simulink model "RespiratorPlantModel"  (R2018b)
settings: Solver=FixedStepAuto  StartTime=0.0  StopTime=30  FixedStep=0.001  MaxStep=0.001  RelTol=1e-3
values from neighbouring files (symbols this model uses):
  BTClockRemoval = 1    [RespiratorPlantModel_init.m]
  Cpoumon = 0.1    [RespiratorPlantModel_init.m]
  Dinttuy = 6    [RespiratorPlantModel_init.m]
  e = 4.5    [RespiratorPlantModel_init.m]
  hlibtuy = 0.05    [RespiratorPlantModel_init.m]
  Patm = 0    [RespiratorPlantModel_init.m]
  Rex = 12.5    [RespiratorPlantModel_init.m]
  Rpoumon = 15    [RespiratorPlantModel_init.m]
  tinsp = 1    [RespiratorPlantModel_init.m]
  X_makair = [0 1.428571429 2.857142857 4.285714286 5.714285714 7.142857143 8.571428571 10 11.42857143 12.85714286 14.28571429 15.71428571 ... (33 elements, 1x33)]    [X_makair.mat]
  Y_makair = [2730.624562 2737.5 2745.890411 2823.971473 2900.599169 3000.432167 3171.512706 3284.514664 3433.346305 3592.109976 3939.708667 4053.269029 ... (33 elements, 1x33)]    [Y_makair.mat]
libraries: simulink x8, simulink_extras x1
settings Model: Creator=FASSI  LastModifiedBy=VITIE
settings SolverCC: AlgebraicLoopSolver=LineSearch

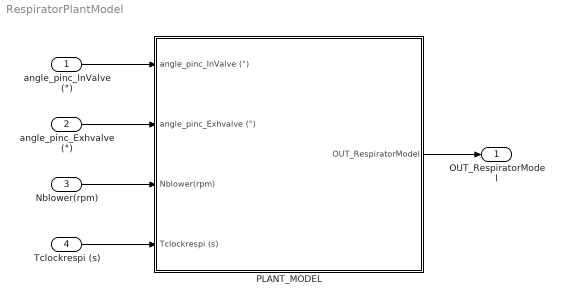
== system RespiratorPlantModel ==
  angle_pinc_InValve (°) : Inport
  angle_pinc_Exhvalve (°) : Inport  Port=2
  Nblower(rpm) : Inport  Port=3
  Tclockrespi (s) : Inport  Port=4
  PLANT_MODEL : Subsystem
  OUT_RespiratorModel : Outport  OutDataTypeStr=Bus: Respirator
  wires:
  angle_pinc_Exhvalve (°)/1 -> PLANT_MODEL/2(angle_pinc_Exhvalve (°))
  angle_pinc_InValve (°)/1 -> PLANT_MODEL/1(angle_pinc_InValve (°))
  Nblower(rpm)/1 -> PLANT_MODEL/3(Nblower(rpm))
  Tclockrespi (s)/1 -> PLANT_MODEL/4(Tclockrespi (s))
  PLANT_MODEL/1(OUT_RespiratorModel) -> OUT_RespiratorModel/1

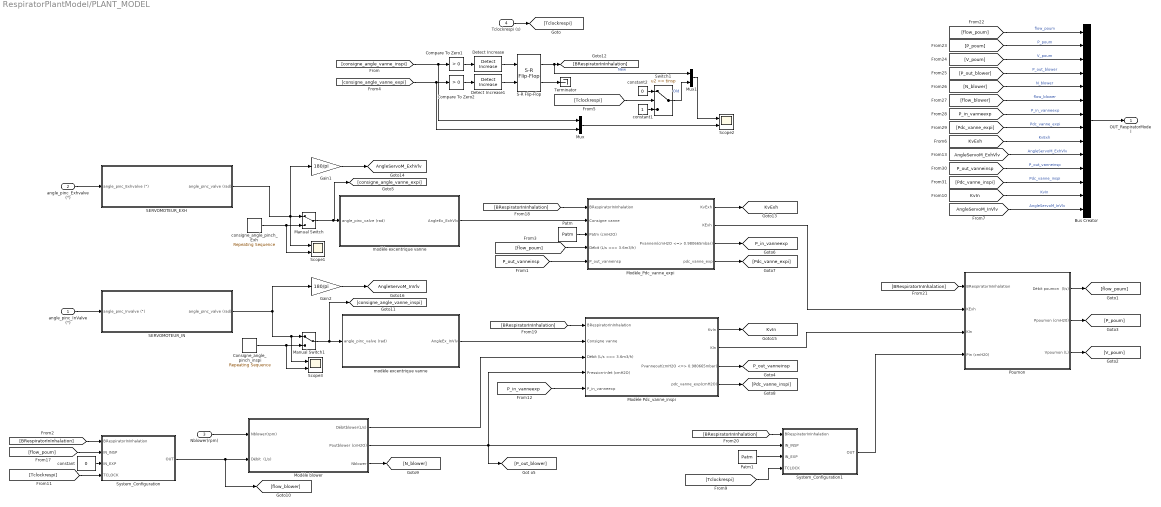
== system RespiratorPlantModel/PLANT_MODEL ==
  angle_pinc_InValve (°) : Inport
  angle_pinc_Exhvalve (°) : Inport  Port=2
  Nblower(rpm) : Inport  Port=3
  Tclockrespi (s) : Inport  Port=4
  Bus Creator : BusCreator  Inputs=14
  Compare To Zero1 : simulink/Logic and Bit Operations/Compare To Zero  relop=>  OutDataTypeStr=boolean
  Compare To Zero2 : simulink/Logic and Bit Operations/Compare To Zero  relop=>  OutDataTypeStr=boolean
  Consigne_angle_pinch_inspi : simulink/Sources/Repeating Sequence  rep_seq_t=X_insp  rep_seq_y=[0 pi pi pi 0 0 0]
  Detect Increase : simulink/Logic and Bit Operations/Detect Increase  vinit=0.0  OutDataTypeStr=boolean
  Detect Increase1 : simulink/Logic and Bit Operations/Detect Increase  vinit=0.0  OutDataTypeStr=boolean
  Gain1 : Gain  Gain=180/pi
  Gain2 : Gain  Gain=180/pi
  Manual Switch : ManualSwitch
  Manual Switch1 : ManualSwitch
  Modèle Pdc_vanne_inspi : Subsystem
  Modèle blower : Subsystem
  Modèle_Pdc_vanne_expi : Subsystem
  Mux : Mux  Inputs=2
  Mux1 : Mux  Inputs=2
  Patm : Constant  Value=Patm
  Patm1 : Constant  Value=Patm
  Poumon : Subsystem
  S-R Flip-Flop : simulink_extras/Flip Flops/S-R Flip-Flop  initial_condition=1
  SERVOMOTEUR_EXH : Subsystem
  SERVOMOTEUR_IN : Subsystem
  Scope1 : Scope  NumInputPorts=2
  Scope2 : Scope  NumInputPorts=2
  Scope3 : Scope  NumInputPorts=2
  Switch1 : Switch  Threshold=tinsp
  System_Configuration : Subsystem
  System_Configuration1 : Subsystem
  Terminator : Terminator
  consigne_angle_pinch_Exh : simulink/Sources/Repeating Sequence  rep_seq_t=X_exp  rep_seq_y=[0 0 0 pi pi 0 0]
  constant : Constant  Value=0
  constant1 : Constant  OutDataTypeStr=boolean
  constant2 : Constant  Value=0  OutDataTypeStr=boolean
  modèle excentrique vanne : Subsystem
  "modèle excentrique vanne " : Subsystem
  OUT_RespiratorModel : Outport
  tag scope: AngleServoM_ExhVlv=global, AngleServoM_InVlv=global, KvExh=global, KvIn=global, P_in_vanneexp=global, P_out_vanneinsp=global
  wires:
  [V_poum] -> Bus Creator/3  "V_poum"
  Compare To Zero1/1 -> Detect Increase/1
  Modèle_Pdc_vanne_expi/2(KExh) -> Poumon/2(KExh)
  System_Configuration/1(OUT) -> [flow_blower], Modèle blower/2(Débit  (L/s))
  Patm/1 -> Modèle_Pdc_vanne_expi/3(Patm (cmH2O))
  [BRespiratorInInhalation] -> System_Configuration1/1(BRespiratorInInhalation)
  [P_in_vanneexp] -> Modèle Pdc_vanne_inspi/5(P_in_vanneexp)
  Compare To Zero2/1 -> Detect Increase1/1
  [BRespiratorInInhalation] -> System_Configuration/1(BRespiratorInInhalation)
  S-R Flip-Flop/1 -> Mux1/1, [BRespiratorInInhalation]  "New"
  System_Configuration1/1(OUT) -> Poumon/4(Pin (cmH20))
  [BRespiratorInInhalation] -> Poumon/1(BRespiratorInInhalation)
  [BRespiratorInInhalation] -> Modèle_Pdc_vanne_expi/1(BRespiratorInInhalation)
  Modèle_Pdc_vanne_expi/4(pdc_vanne_exp) -> [Pdc_vanne_expi]
  [Pdc_vanne_inspi] -> Bus Creator/12  "Pdc_vanne_inspi"
  [consigne_angle_vanne_expi] -> Mux/2, Compare To Zero2/1
  constant/1 -> System_Configuration/3(IN_EXP)
  Patm1/1 -> System_Configuration1/3(IN_EXP)
  Poumon/3(Vpoumon (L)) -> [V_poum]
  Poumon/1(Débit poumon  (l/s)) -> [flow_poum]
  Detect Increase1/1 -> S-R Flip-Flop/2
  "modèle excentrique vanne "/1(AngleEx_InVlv) -> Modèle Pdc_vanne_inspi/2(Consigne vanne)
  [Tclockrespi] -> System_Configuration/4(TCLOCK)
  S-R Flip-Flop/2 -> Terminator/1
  Modèle blower/2(Poutblower (cnH2O)) -> [P_out_blower], System_Configuration1/2(IN_INSP), Modèle Pdc_vanne_inspi/4(Pression-inlet (cmH2O))
  [consigne_angle_vanne_inspi] -> Mux/1, Compare To Zero1/1
  Bus Creator/1 -> OUT_RespiratorModel/1
  [flow_poum] -> Bus Creator/1  "flow_poum"
  [flow_blower] -> Bus Creator/6  "flow_blower"
  [P_out_vanneinsp] -> Modèle_Pdc_vanne_expi/5(P_out_vanneinsp)
  [flow_poum] -> System_Configuration/2(IN_INSP)
  [P_out_vanneinsp] -> Bus Creator/11  "P_out_vanneinsp"
  Detect Increase/1 -> S-R Flip-Flop/1
  Poumon/2(Ppoumon (cmH20)) -> [P_poum]
  Modèle blower/1(Débitblower(L/s)) -> Modèle Pdc_vanne_inspi/3(Débit (L/s <=> 3.6m3/h))
  [Tclockrespi] -> System_Configuration1/4(TCLOCK)
  [flow_poum] -> Modèle_Pdc_vanne_expi/4(Débit (L/s <=> 3.6m3/h))
  modèle excentrique vanne/1(AngleEx_ExhVlv) -> Modèle_Pdc_vanne_expi/2(Consigne vanne)
  [BRespiratorInInhalation] -> Modèle Pdc_vanne_inspi/1(BRespiratorInInhalation)
  [N_blower] -> Bus Creator/5  "N_blower"
  Modèle Pdc_vanne_inspi/2(KIn) -> Poumon/3("KIn ")
  Modèle Pdc_vanne_inspi/4(pdc_vanne_exp(cmH2O)) -> [Pdc_vanne_inspi]
  Modèle_Pdc_vanne_expi/3(Pvannein(cmH2O <=> 0.980665mbar)) -> [P_in_vanneexp]
  Modèle Pdc_vanne_inspi/3(Pvanneout(cmH2O <=> 0.980665mbar)) -> [P_out_vanneinsp]
  Modèle blower/3(Nblower) -> [N_blower]
  [P_out_blower] -> Bus Creator/4  "P_out_blower"
  [P_in_vanneexp] -> Bus Creator/7  "P_in_vanneexp"
  [Pdc_vanne_expi] -> Bus Creator/8  "Pdc_vanne_expi"
  [P_poum] -> Bus Creator/2  "P_poum"
  Nblower(rpm)/1 -> Modèle blower/1(Nblower(rpm))
  Tclockrespi (s)/1 -> [Tclockrespi]
  Mux/1 -> Scope2/2
  [Tclockrespi] -> Switch1/2
  Switch1/1 -> Mux1/2  "Old"
  Mux1/1 -> Scope2/1
  constant1/1 -> Switch1/3
  constant2/1 -> Switch1/1
  angle_pinc_Exhvalve (°)/1 -> SERVOMOTEUR_EXH/1(angle_pinc_Exhvalve (°))
  SERVOMOTEUR_EXH/1(angle_pinc_valve (rad)) -> Scope1/1, Gain1/1, Manual Switch/1
  Manual Switch/1 -> [consigne_angle_vanne_expi], modèle excentrique vanne/1(angle_pinc_valve (rad))
  SERVOMOTEUR_IN/1(angle_pinc_valve (rad)) -> Scope3/1, Manual Switch1/1, Gain2/1
  angle_pinc_InValve (°)/1 -> SERVOMOTEUR_IN/1(angle_pinc_Invalve (°))
  Consigne_angle_pinch_inspi/1 -> Scope3/2, Manual Switch1/2
  Manual Switch1/1 -> [consigne_angle_vanne_inspi], "modèle excentrique vanne "/1(angle_pinc_valve (rad))
  [KvExh] -> Bus Creator/9  "KvExh"
  [AngleServoM_ExhVlv] -> Bus Creator/10  "AngleServoM_ExhVlv"
  [AngleServoM_InVlv] -> Bus Creator/14  "AngleServoM_InVlv"
  [KvIn] -> Bus Creator/13  "KvIn"
  consigne_angle_pinch_Exh/1 -> Scope1/2, Manual Switch/2
  Gain1/1 -> [AngleServoM_ExhVlv]
  Gain2/1 -> [AngleServoM_InVlv]
  Modèle_Pdc_vanne_expi/1(KvExh) -> [KvExh]
  Modèle Pdc_vanne_inspi/1(KvIn) -> [KvIn]

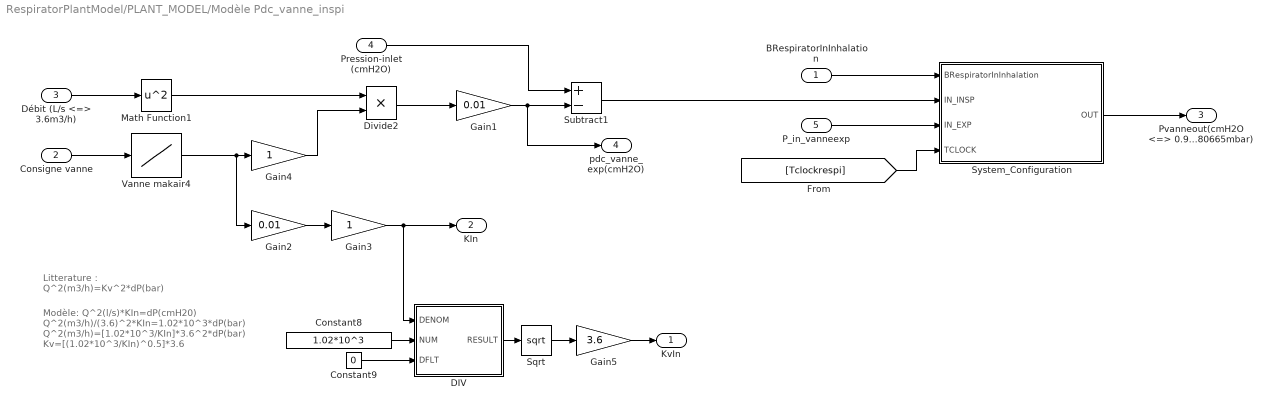
== system RespiratorPlantModel/PLANT_MODEL/Modèle Pdc_vanne_inspi ==
  note: Litterature :
      | Q^2(m3/h)=Kv^2*dP(bar)
  note: Modèle:
      | Q^2(l/s)*KIn=dP(cmH20)
      | Q^2(m3/h)/(3.6)^2*KIn=1.02*10^3*dP(bar)
      | Q^2(m3/h)=[1.02*10^3/KIn]*3.6^2*dP(bar)
      |
      | Kv=[(1.02*10^3/KIn)^0.5]*3.6
  BRespiratorInInhalation : Inport
  Consigne vanne : Inport  Port=2
  Débit (L/s <=> 3.6m3/h) : Inport  Port=3
  Pression-inlet (cmH2O) : Inport  Port=4
  P_in_vanneexp : Inport  Port=5
  Constant8 : Constant  Value=1.02*10^3
  Constant9 : Constant  Value=0
  DIV : Subsystem  mask(DIV){}
      mask help: This block executes a division with protection for division by 0.
      mask Display: disp('DIV')
  Divide2 : Product  Inputs=**
  Gain1 : Gain  Gain=0.01
  Gain2 : Gain  Gain=0.01
  Gain3 : Gain
  Gain4 : Gain
  Gain5 : Gain  Gain=3.6
  Math Function1 : Math  Operator=square  SaturateOnIntegerOverflow=on
  Sqrt : Sqrt  SaturateOnIntegerOverflow=on
  Subtract1 : Sum  Inputs=+-
  System_Configuration : Subsystem
  Vanne makair4 : Lookup_n-D  NumberOfTableDimensions=1  LookupTableObject=vanne_makair  BreakpointsForDimension1=X_makair  Table=Y_makair  InternalRulePriority=Speed  RndMeth=Simplest  InputSameDT=on
  KvIn : Outport
  KIn : Outport  Port=2
  Pvanneout(cmH2O <=> 0.980665mbar) : Outport  Port=3
  pdc_vanne_exp(cmH2O) : Outport  Port=4
  wires:
  Math Function1/1 -> Divide2/1
  Vanne makair4/1 -> Gain2/1, Gain4/1
  Débit (L/s <=> 3.6m3/h)/1 -> Math Function1/1
  Consigne vanne/1 -> Vanne makair4/1
  Divide2/1 -> Gain1/1
  Pression-inlet (cmH2O)/1 -> Subtract1/1
  Gain1/1 -> pdc_vanne_exp(cmH2O)/1, Subtract1/2
  Gain2/1 -> Gain3/1
  System_Configuration/1(OUT) -> Pvanneout(cmH2O <=> 0.980665mbar)/1
  Gain4/1 -> Divide2/2
  P_in_vanneexp/1 -> System_Configuration/3(IN_EXP)
  [Tclockrespi] -> System_Configuration/4(TCLOCK)
  Subtract1/1 -> System_Configuration/2(IN_INSP)
  BRespiratorInInhalation/1 -> System_Configuration/1(BRespiratorInInhalation)
  Gain5/1 -> KvIn/1
  Constant9/1 -> DIV/3(DFLT)
  Gain3/1 -> DIV/1(DENOM), KIn/1
  Sqrt/1 -> Gain5/1
  Constant8/1 -> DIV/2(NUM)
  DIV/1(RESULT) -> Sqrt/1

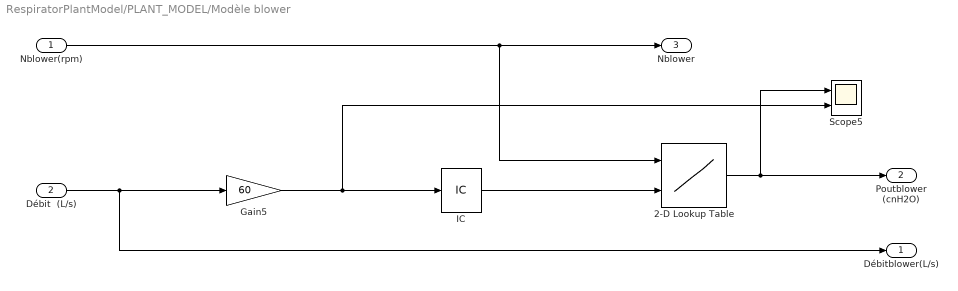
== system RespiratorPlantModel/PLANT_MODEL/Modèle blower ==
  Nblower(rpm) : Inport
  Débit  (L/s) : Inport  Port=2
  2-D Lookup Table : Lookup_n-D  BreakpointsForDimension1=[0,30000,41000,54000]  BreakpointsForDimension2=[0,15,30,50,80,100,120,140,160]  Table=reshape([0,32.2,60.6,103.8,0,31.8,59.6,103.5,0,31,59.1,102.2,0,29.2,56.5,100,0,24.8,52.4,93.7,0,20,48.2,88.8,0,15.2,43.8,82.8,0,9.1,36.3,77.2,0,1.4,29.1,71.6],4,9)  ExtrapMethod=Clip  InternalRulePriority=Speed  RndMeth=Simplest  InputSameDT=on
  Gain5 : Gain  Gain=60
  IC : InitialCondition  Value=0
  Scope5 : Scope  NumInputPorts=2
  Débitblower(L/s) : Outport
  Poutblower (cnH2O) : Outport  Port=2
  Nblower : Outport  Port=3
  wires:
  Gain5/1 -> Scope5/2, IC/1
  Nblower(rpm)/1 -> 2-D Lookup Table/1, Nblower/1
  Débit  (L/s)/1 -> Débitblower(L/s)/1, Gain5/1
  2-D Lookup Table/1 -> Scope5/1, Poutblower (cnH2O)/1
  IC/1 -> 2-D Lookup Table/2

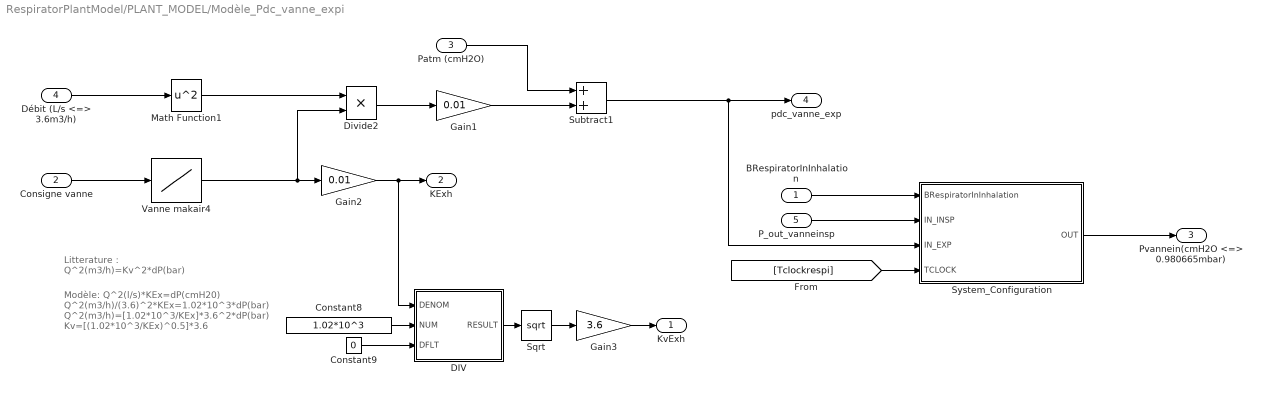
== system RespiratorPlantModel/PLANT_MODEL/Modèle_Pdc_vanne_expi ==
  note: Litterature :
      | Q^2(m3/h)=Kv^2*dP(bar)
  note: Modèle:
      | Q^2(l/s)*KEx=dP(cmH20)
      | Q^2(m3/h)/(3.6)^2*KEx=1.02*10^3*dP(bar)
      | Q^2(m3/h)=[1.02*10^3/KEx]*3.6^2*dP(bar)
      |
      | Kv=[(1.02*10^3/KEx)^0.5]*3.6
  BRespiratorInInhalation : Inport
  Consigne vanne : Inport  Port=2
  Patm (cmH2O) : Inport  Port=3
  Débit (L/s <=> 3.6m3/h) : Inport  Port=4
  P_out_vanneinsp : Inport  Port=5
  Constant8 : Constant  Value=1.02*10^3
  Constant9 : Constant  Value=0
  DIV : Subsystem  mask(DIV){}
      mask help: This block executes a division with protection for division by 0.
      mask Display: disp('DIV')
  Divide2 : Product  Inputs=**
  Gain1 : Gain  Gain=0.01
  Gain2 : Gain  Gain=0.01
  Gain3 : Gain  Gain=3.6
  Math Function1 : Math  Operator=square  SaturateOnIntegerOverflow=on
  Sqrt : Sqrt  SaturateOnIntegerOverflow=on
  Subtract1 : Sum
  System_Configuration : Subsystem
  Vanne makair4 : Lookup_n-D  NumberOfTableDimensions=1  LookupTableObject=vanne_makair  BreakpointsForDimension1=X_makair  Table=Y_makair  InternalRulePriority=Speed  RndMeth=Simplest  InputSameDT=on
  KvExh : Outport
  KExh : Outport  Port=2
  Pvannein(cmH2O <=> 0.980665mbar) : Outport  Port=3
  pdc_vanne_exp : Outport  Port=4
  wires:
  Math Function1/1 -> Divide2/1
  Débit (L/s <=> 3.6m3/h)/1 -> Math Function1/1
  Consigne vanne/1 -> Vanne makair4/1
  Divide2/1 -> Gain1/1
  Patm (cmH2O)/1 -> Subtract1/1
  Gain1/1 -> Subtract1/2
  Gain2/1 -> DIV/1(DENOM), KExh/1
  Subtract1/1 -> System_Configuration/3(IN_EXP), pdc_vanne_exp/1
  [Tclockrespi] -> System_Configuration/4(TCLOCK)
  BRespiratorInInhalation/1 -> System_Configuration/1(BRespiratorInInhalation)
  System_Configuration/1(OUT) -> Pvannein(cmH2O <=> 0.980665mbar)/1
  P_out_vanneinsp/1 -> System_Configuration/2(IN_INSP)
  Constant8/1 -> DIV/2(NUM)
  Vanne makair4/1 -> Gain2/1, Divide2/2
  Constant9/1 -> DIV/3(DFLT)
  DIV/1(RESULT) -> Sqrt/1
  Sqrt/1 -> Gain3/1
  Gain3/1 -> KvExh/1

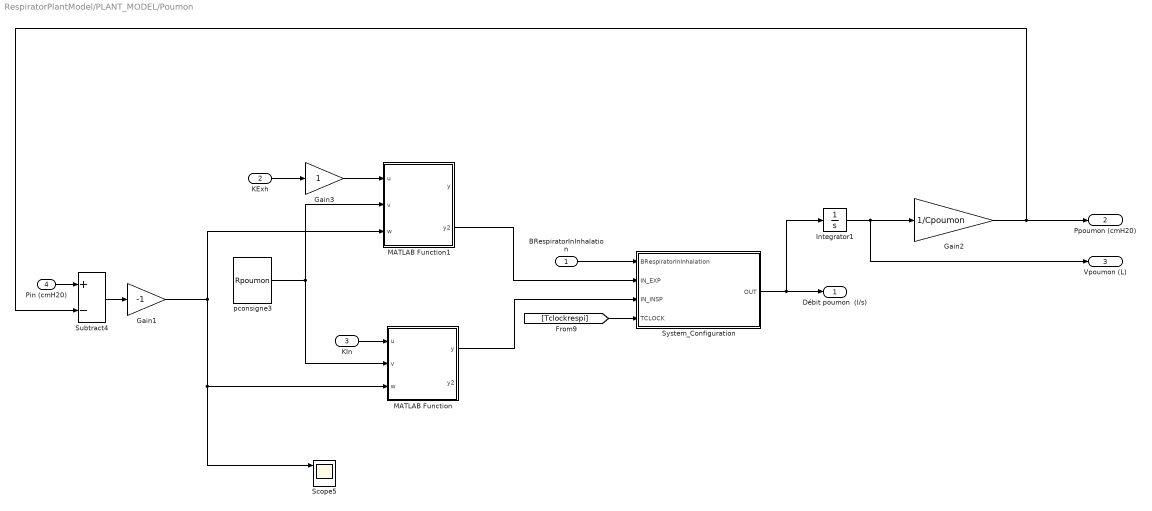
== system RespiratorPlantModel/PLANT_MODEL/Poumon ==
  BRespiratorInInhalation : Inport
  KExh : Inport  Port=2
  "KIn " : Inport  Port=3
  Pin (cmH20) : Inport  Port=4
  Gain1 : Gain  Gain=-1
  Gain2 : Gain  Gain=1/Cpoumon
  Gain3 : Gain
  Integrator1 : Integrator
  MATLAB Function : MATLAB Function  TreatAsAtomicUnit=on
  MATLAB Function1 : MATLAB Function  TreatAsAtomicUnit=on
  Scope5 : Scope  NumInputPorts=3
  Subtract4 : Sum  Inputs=+-
  System_Configuration : Subsystem
  pconsigne3 : Constant  Value=Rpoumon
  Débit poumon  (l/s) : Outport
  Ppoumon (cmH20) : Outport  Port=2
  Vpoumon (L) : Outport  Port=3
  wires:
  Gain2/1 -> Subtract4/2, Ppoumon (cmH20)/1
  Pin (cmH20)/1 -> Subtract4/1
  pconsigne3/1 -> MATLAB Function1/2(v), MATLAB Function/2(v)
  Gain1/1 -> MATLAB Function1/3(w), MATLAB Function/3(w), Scope5/1
  "KIn "/1 -> MATLAB Function/1(u)
  Integrator1/1 -> Vpoumon (L)/1, Gain2/1
  MATLAB Function/1(y) -> System_Configuration/3(IN_INSP)
  Subtract4/1 -> Gain1/1
  KExh/1 -> Gain3/1
  Gain3/1 -> MATLAB Function1/1(u)
  System_Configuration/1(OUT) -> Integrator1/1, Débit poumon  (l/s)/1
  MATLAB Function1/2(y2) -> System_Configuration/2(IN_EXP)
  [Tclockrespi] -> System_Configuration/4(TCLOCK)
  BRespiratorInInhalation/1 -> System_Configuration/1(BRespiratorInInhalation)

== system RespiratorPlantModel/PLANT_MODEL/SERVOMOTEUR_EXH ==
  angle_pinc_Exhvalve (°) : Inport
  Gain : Gain  Gain=pi/180
  Rate Limiter Dynamic : simulink/Discontinuities/Rate Limiter Dynamic
      settings: SourceProductName=Simulink
  Slope : Constant  Value=pi/0.150
  Slope1 : Constant  Value=-pi/0.150
  angle_pinc_valve (rad) : Outport
  wires:
  angle_pinc_Exhvalve (°)/1 -> Gain/1
  Rate Limiter Dynamic/1 -> angle_pinc_valve (rad)/1
  Gain/1 -> Rate Limiter Dynamic/2
  Slope/1 -> Rate Limiter Dynamic/1
  Slope1/1 -> Rate Limiter Dynamic/3

== system RespiratorPlantModel/PLANT_MODEL/SERVOMOTEUR_IN ==
  angle_pinc_Invalve (°) : Inport
  Gain : Gain  Gain=pi/180
  Rate Limiter Dynamic : simulink/Discontinuities/Rate Limiter Dynamic
      settings: SourceProductName=Simulink
  Slope : Constant  Value=pi/0.150
  Slope1 : Constant  Value=-pi/0.150
  angle_pinc_valve (rad) : Outport
  wires:
  Rate Limiter Dynamic/1 -> angle_pinc_valve (rad)/1
  angle_pinc_Invalve (°)/1 -> Gain/1
  Slope1/1 -> Rate Limiter Dynamic/3
  Slope/1 -> Rate Limiter Dynamic/1
  Gain/1 -> Rate Limiter Dynamic/2

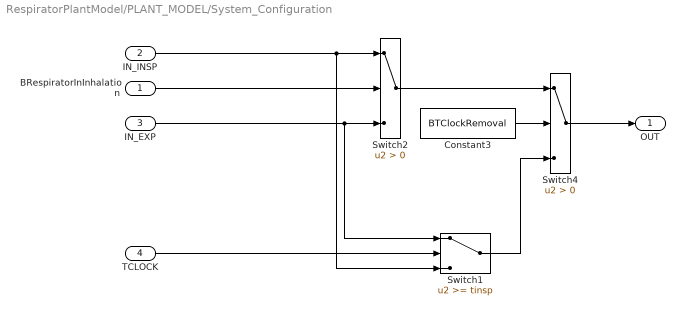
== system RespiratorPlantModel/PLANT_MODEL/System_Configuration ==
  BRespiratorInInhalation : Inport
  IN_INSP : Inport  Port=2
  IN_EXP : Inport  Port=3
  TCLOCK : Inport  Port=4
  Constant3 : Constant  Value=BTClockRemoval
  Switch1 : Switch  Threshold=tinsp
  Switch2 : Switch  Criteria=u2 > Threshold
      settings: AttributesFormatString=%<Criteria>
  Switch4 : Switch  Criteria=u2 > Threshold
      settings: AttributesFormatString=%<Criteria>
  OUT : Outport
  wires:
  Constant3/1 -> Switch4/2
  Switch2/1 -> Switch4/1
  Switch1/1 -> Switch4/3
  TCLOCK/1 -> Switch1/2
  Switch4/1 -> OUT/1
  IN_INSP/1 -> Switch1/3, Switch2/1
  BRespiratorInInhalation/1 -> Switch2/2
  IN_EXP/1 -> Switch1/1, Switch2/3

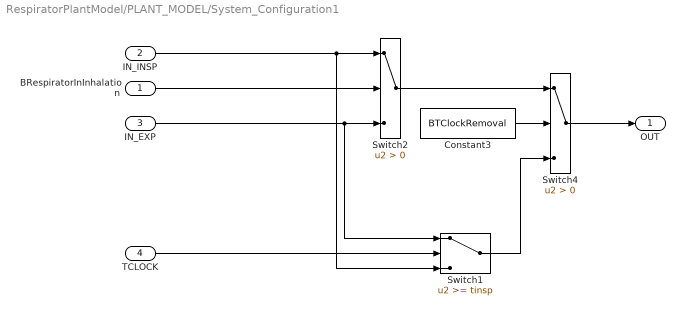
== system RespiratorPlantModel/PLANT_MODEL/System_Configuration1 ==
  BRespiratorInInhalation : Inport
  IN_INSP : Inport  Port=2
  IN_EXP : Inport  Port=3
  TCLOCK : Inport  Port=4
  Constant3 : Constant  Value=BTClockRemoval
  Switch1 : Switch  Threshold=tinsp
  Switch2 : Switch  Criteria=u2 > Threshold
      settings: AttributesFormatString=%<Criteria>
  Switch4 : Switch  Criteria=u2 > Threshold
      settings: AttributesFormatString=%<Criteria>
  OUT : Outport
  wires:
  Constant3/1 -> Switch4/2
  Switch2/1 -> Switch4/1
  Switch1/1 -> Switch4/3
  TCLOCK/1 -> Switch1/2
  Switch4/1 -> OUT/1
  IN_INSP/1 -> Switch1/3, Switch2/1
  BRespiratorInInhalation/1 -> Switch2/2
  IN_EXP/1 -> Switch1/1, Switch2/3

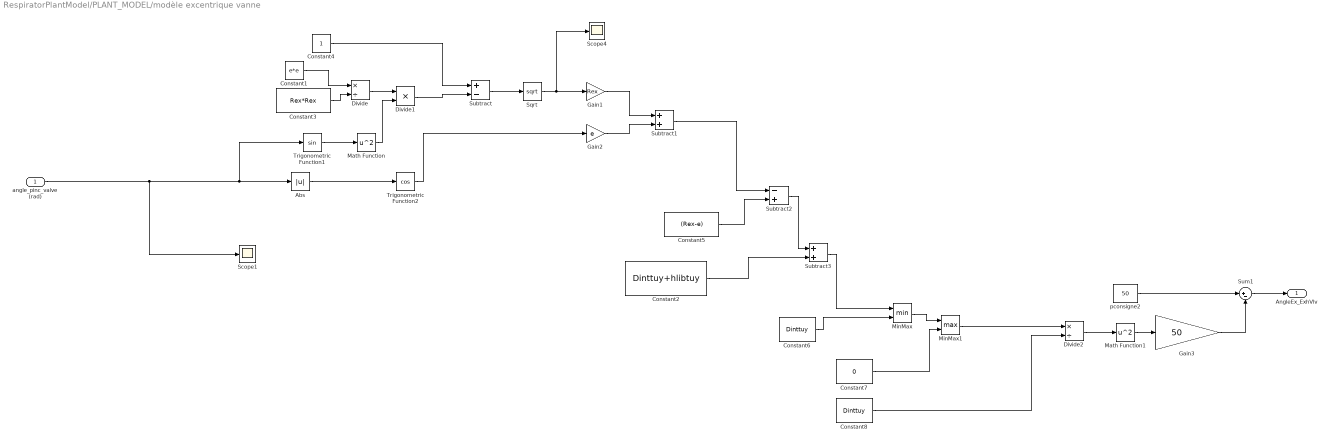
== system RespiratorPlantModel/PLANT_MODEL/modèle excentrique vanne ==
  angle_pinc_valve (rad) : Inport
  Abs : Abs
  Constant1 : Constant  Value=e*e
  Constant2 : Constant  Value=Dinttuy+hlibtuy
  Constant3 : Constant  Value=Rex*Rex
  Constant4 : Constant
  Constant5 : Constant  Value=(Rex-e)
  Constant6 : Constant  Value=Dinttuy
  Constant7 : Constant  Value=0
  Constant8 : Constant  Value=Dinttuy
  Divide : Product  Inputs=*/
  Divide1 : Product  Inputs=**
  Divide2 : Product  Inputs=*/
  Gain1 : Gain  Gain=Rex
  Gain2 : Gain  Gain=e
  Gain3 : Gain  Gain=50
  Math Function : Math  Operator=square  SaturateOnIntegerOverflow=on
  Math Function1 : Math  Operator=square  SaturateOnIntegerOverflow=on
  MinMax : MinMax  Inputs=2
  MinMax1 : MinMax  Function=max  Inputs=2
  Scope1 : Scope
  Scope4 : Scope
  Sqrt : Sqrt  SaturateOnIntegerOverflow=on
  Subtract : Sum  Inputs=+-
  Subtract1 : Sum
  Subtract2 : Sum  Inputs=-+
  Subtract3 : Sum
  Sum1 : Sum  Inputs=|+-
  Trigonometric Function1 : Trigonometry
  Trigonometric Function2 : Trigonometry  Operator=cos
  pconsigne2 : Constant  Value=50
  AngleEx_ExhVlv : Outport
  wires:
  Constant1/1 -> Divide/1
  Trigonometric Function1/1 -> Math Function/1
  Constant4/1 -> Subtract/1
  Divide1/1 -> Subtract/2
  Subtract/1 -> Sqrt/1
  Constant3/1 -> Divide/2
  Subtract1/1 -> Subtract2/1
  Gain1/1 -> Subtract1/1
  Abs/1 -> Trigonometric Function2/1
  Sqrt/1 -> Scope4/1, Gain1/1
  Math Function/1 -> Divide1/2
  Gain2/1 -> Subtract1/2
  angle_pinc_valve (rad)/1 -> Scope1/1, Trigonometric Function1/1, Abs/1
  Divide/1 -> Divide1/1
  Trigonometric Function2/1 -> Gain2/1
  Constant5/1 -> Subtract2/2
  Constant2/1 -> Subtract3/2
  Subtract2/1 -> Subtract3/1
  Constant6/1 -> MinMax/2
  Subtract3/1 -> MinMax/1
  MinMax/1 -> MinMax1/1
  Constant7/1 -> MinMax1/2
  MinMax1/1 -> Divide2/1
  Constant8/1 -> Divide2/2
  Divide2/1 -> Math Function1/1
  Sum1/1 -> AngleEx_ExhVlv/1
  Gain3/1 -> Sum1/2
  pconsigne2/1 -> Sum1/1
  Math Function1/1 -> Gain3/1

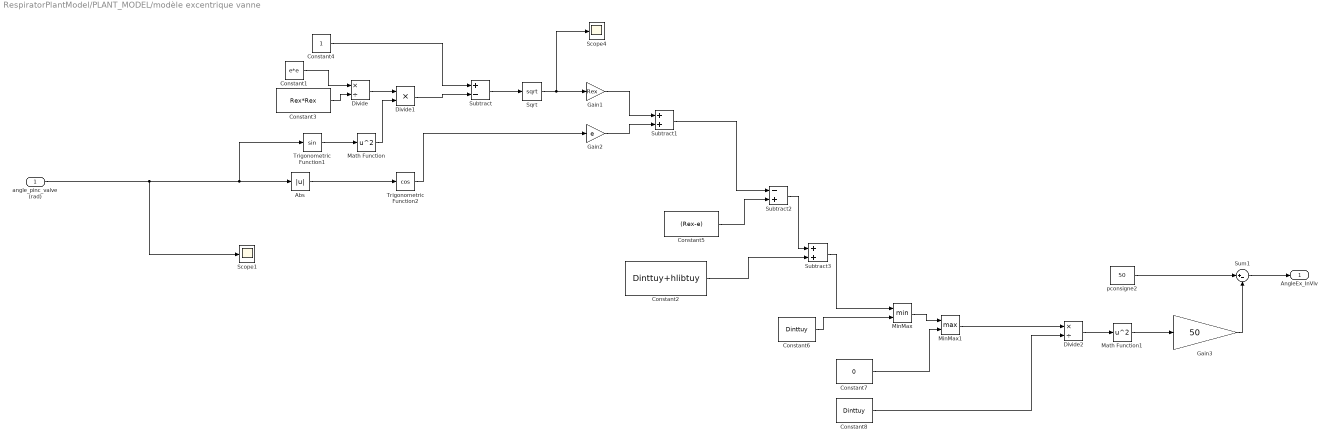
== system RespiratorPlantModel/PLANT_MODEL/modèle excentrique vanne  ==
  angle_pinc_valve (rad) : Inport
  Abs : Abs
  Constant1 : Constant  Value=e*e
  Constant2 : Constant  Value=Dinttuy+hlibtuy
  Constant3 : Constant  Value=Rex*Rex
  Constant4 : Constant
  Constant5 : Constant  Value=(Rex-e)
  Constant6 : Constant  Value=Dinttuy
  Constant7 : Constant  Value=0
  Constant8 : Constant  Value=Dinttuy
  Divide : Product  Inputs=*/
  Divide1 : Product  Inputs=**
  Divide2 : Product  Inputs=*/
  Gain1 : Gain  Gain=Rex
  Gain2 : Gain  Gain=e
  Gain3 : Gain  Gain=50
  Math Function : Math  Operator=square  SaturateOnIntegerOverflow=on
  Math Function1 : Math  Operator=square  SaturateOnIntegerOverflow=on
  MinMax : MinMax  Inputs=2
  MinMax1 : MinMax  Function=max  Inputs=2
  Scope1 : Scope
  Scope4 : Scope
  Sqrt : Sqrt  SaturateOnIntegerOverflow=on
  Subtract : Sum  Inputs=+-
  Subtract1 : Sum
  Subtract2 : Sum  Inputs=-+
  Subtract3 : Sum
  Sum1 : Sum  Inputs=|+-
  Trigonometric Function1 : Trigonometry
  Trigonometric Function2 : Trigonometry  Operator=cos
  pconsigne2 : Constant  Value=50
  AngleEx_InVlv : Outport
  wires:
  Constant1/1 -> Divide/1
  Trigonometric Function1/1 -> Math Function/1
  Constant4/1 -> Subtract/1
  Divide1/1 -> Subtract/2
  Subtract/1 -> Sqrt/1
  Constant3/1 -> Divide/2
  Subtract1/1 -> Subtract2/1
  Gain1/1 -> Subtract1/1
  Abs/1 -> Trigonometric Function2/1
  Sqrt/1 -> Scope4/1, Gain1/1
  Math Function/1 -> Divide1/2
  Gain2/1 -> Subtract1/2
  angle_pinc_valve (rad)/1 -> Scope1/1, Trigonometric Function1/1, Abs/1
  Divide/1 -> Divide1/1
  Trigonometric Function2/1 -> Gain2/1
  Constant5/1 -> Subtract2/2
  Constant2/1 -> Subtract3/2
  Subtract2/1 -> Subtract3/1
  Constant6/1 -> MinMax/2
  Subtract3/1 -> MinMax/1
  MinMax/1 -> MinMax1/1
  Constant7/1 -> MinMax1/2
  MinMax1/1 -> Divide2/1
  Constant8/1 -> Divide2/2
  Divide2/1 -> Math Function1/1
  Sum1/1 -> AngleEx_InVlv/1
  Gain3/1 -> Sum1/2
  pconsigne2/1 -> Sum1/1
  Math Function1/1 -> Gain3/1

== system RespiratorPlantModel/PLANT_MODEL/Modèle Pdc_vanne_inspi/DIV ==
  DENOM : Inport
  NUM : Inport  Port=2
  DFLT : Inport  Port=3
  Action_Else : Subsystem  TreatAsAtomicUnit=on
  Action_If : Subsystem  TreatAsAtomicUnit=on
  If : If  IfExpression=u1 ~= 0
  Merge : Merge
  RESULT : Outport
  wires:
  Merge/1 -> RESULT/1
  Action_Else/1(RESULT) -> Merge/2
  Action_If/1(RESULT) -> Merge/1
  If/2 -> Action_Else/Action
  DFLT/1 -> Action_Else/1(DFLT)
  DENOM/1 -> If/1, Action_If/2(DENOM)
  NUM/1 -> Action_If/1(NUM)
  If/1 -> Action_If/Action

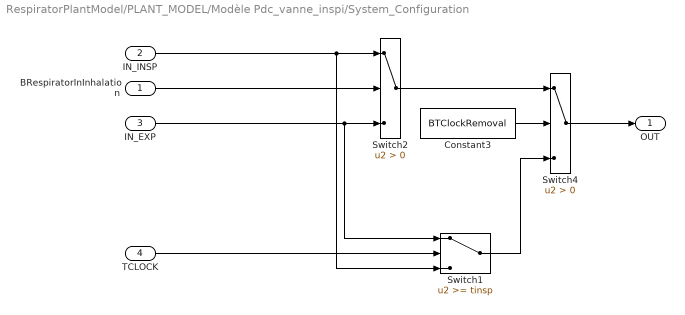
== system RespiratorPlantModel/PLANT_MODEL/Modèle Pdc_vanne_inspi/System_Configuration ==
  BRespiratorInInhalation : Inport
  IN_INSP : Inport  Port=2
  IN_EXP : Inport  Port=3
  TCLOCK : Inport  Port=4
  Constant3 : Constant  Value=BTClockRemoval
  Switch1 : Switch  Threshold=tinsp
  Switch2 : Switch  Criteria=u2 > Threshold
      settings: AttributesFormatString=%<Criteria>
  Switch4 : Switch  Criteria=u2 > Threshold
      settings: AttributesFormatString=%<Criteria>
  OUT : Outport
  wires:
  Constant3/1 -> Switch4/2
  Switch2/1 -> Switch4/1
  Switch1/1 -> Switch4/3
  TCLOCK/1 -> Switch1/2
  Switch4/1 -> OUT/1
  IN_INSP/1 -> Switch1/3, Switch2/1
  BRespiratorInInhalation/1 -> Switch2/2
  IN_EXP/1 -> Switch1/1, Switch2/3

== system RespiratorPlantModel/PLANT_MODEL/Modèle_Pdc_vanne_expi/DIV ==
  DENOM : Inport
  NUM : Inport  Port=2
  DFLT : Inport  Port=3
  Action_Else : Subsystem  TreatAsAtomicUnit=on
  Action_If : Subsystem  TreatAsAtomicUnit=on
  If : If  IfExpression=u1 ~= 0
  Merge : Merge
  RESULT : Outport
  wires:
  Merge/1 -> RESULT/1
  Action_Else/1(RESULT) -> Merge/2
  Action_If/1(RESULT) -> Merge/1
  If/2 -> Action_Else/Action
  DFLT/1 -> Action_Else/1(DFLT)
  DENOM/1 -> If/1, Action_If/2(DENOM)
  NUM/1 -> Action_If/1(NUM)
  If/1 -> Action_If/Action

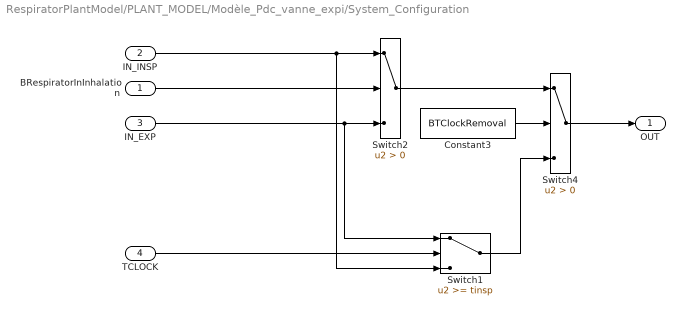
== system RespiratorPlantModel/PLANT_MODEL/Modèle_Pdc_vanne_expi/System_Configuration ==
  BRespiratorInInhalation : Inport
  IN_INSP : Inport  Port=2
  IN_EXP : Inport  Port=3
  TCLOCK : Inport  Port=4
  Constant3 : Constant  Value=BTClockRemoval
  Switch1 : Switch  Threshold=tinsp
  Switch2 : Switch  Criteria=u2 > Threshold
      settings: AttributesFormatString=%<Criteria>
  Switch4 : Switch  Criteria=u2 > Threshold
      settings: AttributesFormatString=%<Criteria>
  OUT : Outport
  wires:
  Constant3/1 -> Switch4/2
  Switch2/1 -> Switch4/1
  Switch1/1 -> Switch4/3
  TCLOCK/1 -> Switch1/2
  Switch4/1 -> OUT/1
  IN_INSP/1 -> Switch1/3, Switch2/1
  BRespiratorInInhalation/1 -> Switch2/2
  IN_EXP/1 -> Switch1/1, Switch2/3

== system RespiratorPlantModel/PLANT_MODEL/Poumon/System_Configuration ==
  BRespiratorInInhalation : Inport
  IN_EXP : Inport  Port=2
  IN_INSP : Inport  Port=3
  TCLOCK : Inport  Port=4
  Constant3 : Constant  Value=BTClockRemoval
  Switch1 : Switch  Threshold=tinsp
  Switch2 : Switch  Criteria=u2 > Threshold
      settings: AttributesFormatString=%<Criteria>
  Switch4 : Switch  Criteria=u2 > Threshold
      settings: AttributesFormatString=%<Criteria>
  OUT : Outport
  wires:
  Constant3/1 -> Switch4/2
  Switch2/1 -> Switch4/1
  Switch1/1 -> Switch4/3
  TCLOCK/1 -> Switch1/2
  Switch4/1 -> OUT/1
  IN_INSP/1 -> Switch1/3, Switch2/1
  BRespiratorInInhalation/1 -> Switch2/2
  IN_EXP/1 -> Switch1/1, Switch2/3

== system RespiratorPlantModel/PLANT_MODEL/Modèle Pdc_vanne_inspi/DIV/Action_Else ==
  DFLT : Inport
  Action Port : ActionPort
  Signal Conversion : SignalConversion  OverrideOpt=off
  RESULT : Outport
  wires:
  Signal Conversion/1 -> RESULT/1
  DFLT/1 -> Signal Conversion/1

== system RespiratorPlantModel/PLANT_MODEL/Modèle Pdc_vanne_inspi/DIV/Action_If ==
  NUM : Inport
  DENOM : Inport  Port=2
  Action Port : ActionPort
  Ideal gas law2 : Product  Inputs=*/
  RESULT : Outport
  wires:
  DENOM/1 -> Ideal gas law2/2
  Ideal gas law2/1 -> RESULT/1
  NUM/1 -> Ideal gas law2/1

== system RespiratorPlantModel/PLANT_MODEL/Modèle_Pdc_vanne_expi/DIV/Action_Else ==
  DFLT : Inport
  Action Port : ActionPort
  Signal Conversion : SignalConversion  OverrideOpt=off
  RESULT : Outport
  wires:
  Signal Conversion/1 -> RESULT/1
  DFLT/1 -> Signal Conversion/1

== system RespiratorPlantModel/PLANT_MODEL/Modèle_Pdc_vanne_expi/DIV/Action_If ==
  NUM : Inport
  DENOM : Inport  Port=2
  Action Port : ActionPort
  Ideal gas law2 : Product  Inputs=*/
  RESULT : Outport
  wires:
  DENOM/1 -> Ideal gas law2/2
  Ideal gas law2/1 -> RESULT/1
  NUM/1 -> Ideal gas law2/1

== matlab function RespiratorPlantModel/PLANT_MODEL/Poumon/MATLAB Function1 ==
  data: u input; y output; v input; w input; y2 output
function [y,y2] = fcn(u,v,w)
vec=roots([-u v w]);
if vec(1,1)>0
    y = real(vec(1,1));
    y2= real(vec(2,1));
else
y = real(vec(2,1));
y2=real(vec(1,1));
end;

== matlab function RespiratorPlantModel/PLANT_MODEL/Poumon/MATLAB Function ==
  data: u input; y output; v input; w input; y2 output
function [y,y2] = fcn(u,v,w)
vec=roots([u v w]);
if vec(1,1)>0
    y = real(vec(1,1));
    y2= real(vec(2,1));
else
y = real(vec(2,1));
y2=real(vec(1,1));
end;
